simulink model "newscalemodel"  (R2019b)
settings: Solver=VariableStepAuto  StartTime=0.0  StopTime=30  RelTol=1e-3
undefined symbols (not defined in the file or in its folder): scalemodelstatefunction
settings Model: Creator=Vlad  LastModifiedBy=Vlad

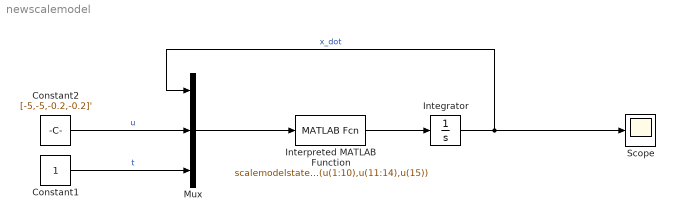
== system newscalemodel ==
  Constant1 : Constant
  Constant2 : Constant  Value=[-5,-5,-0.2,-0.2]'
  Integrator : Integrator
  Interpreted MATLAB Function : MATLABFcn  MATLABFcn=scalemodelstatefunction(u(1:10),u(11:14),u(15))  OutputDimensions=10
  Mux : Mux  Inputs=3
  Scope : Scope
  wires:
  Mux/1 -> Interpreted MATLAB Function/1
  Constant1/1 -> Mux/3  "t"
  Constant2/1 -> Mux/2  "u"
  Interpreted MATLAB Function/1 -> Integrator/1
  Integrator/1 -> Scope/1, Mux/1  "x_dot"
